simulink model "PASTd"  (R2024b)
settings: Solver=VariableStepAuto  StartTime=0.0  StopTime=10.0  RelTol=1e-3
model workspace (MAT data in the model file):
  w0 = 1
undefined symbols (not defined in the file or in its folder): magnitude
libraries: matrix_library x2
settings Model: ParameterArgumentNames=w0  Creator=yingwan  LastModifiedBy=yingwan
settings ConfigComp: CovBoundaryAbsTol=1.0e-5

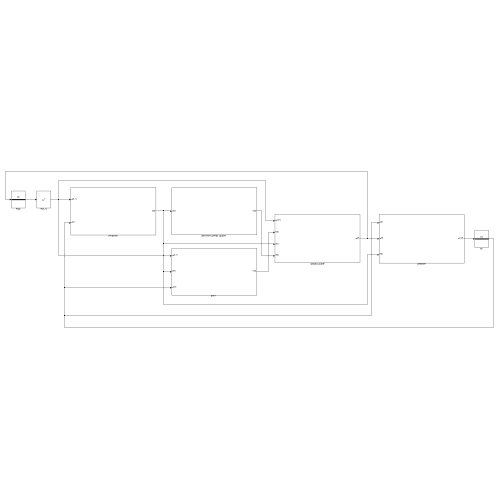
[thumbnail: Simulink's stored preview of the top-level diagram]
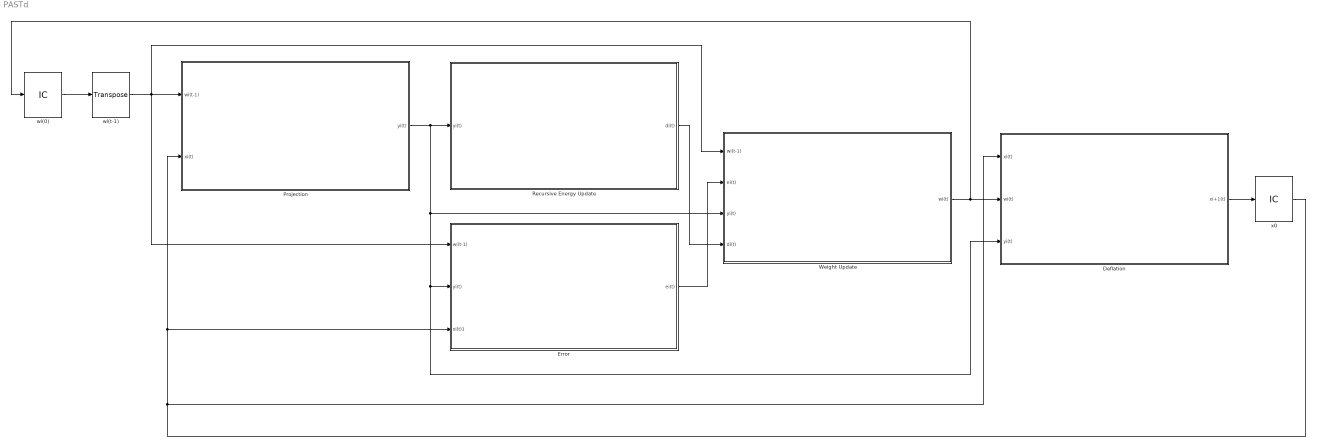
== system PASTd ==
  " Deflation" : Subsystem
  " Weight Update" : Subsystem
  "Error   " : Subsystem
  Projection : Subsystem
  "Recursive Energy Update  " : Subsystem
  wi(0) : InitialCondition
  wi(t-1) : matrix_library/Transpose
  x0 : InitialCondition
  wires:
  Projection/1(yi(t)) -> " Weight Update"/3(yi(t)), " Deflation"/3(yi(t)), "Error   "/2(yi(t)), "Recursive Energy Update  "/1(yi(t))
  wi(t-1)/1 -> "Error   "/1(wi(t-1)), Projection/1(wi(t-1)), " Weight Update"/1(wi(t-1))
  x0/1 -> Projection/2(xi(t)), "Error   "/3(xi(t)1), " Deflation"/1(xi(t))
  " Weight Update"/1(wi(t)) -> wi(0)/1, " Deflation"/2(wi(t))
  "Error   "/1(ei(t)) -> " Weight Update"/2(ei(t))
  "Recursive Energy Update  "/1(di(t)) -> " Weight Update"/4(di(t))
  wi(0)/1 -> wi(t-1)/1
  " Deflation"/1(xi+1(t)) -> x0/1

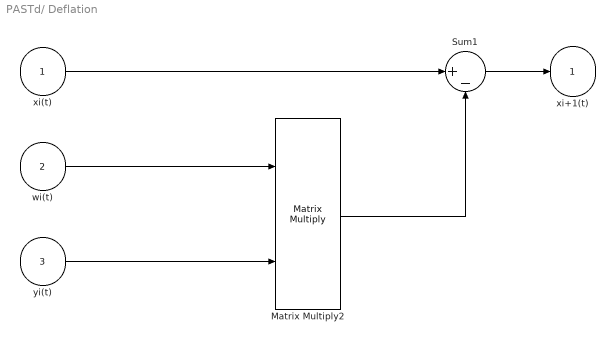
== system PASTd/ Deflation ==
  xi(t) : Inport
  wi(t) : Inport  Port=2
  yi(t) : Inport  Port=3
  Matrix Multiply2 : Product  Multiplication=Matrix(*)
  Sum1 : Sum  Inputs=|+-
  xi+1(t) : Outport
  wires:
  wi(t)/1 -> Matrix Multiply2/1
  yi(t)/1 -> Matrix Multiply2/2
  xi(t)/1 -> Sum1/1
  Matrix Multiply2/1 -> Sum1/2
  Sum1/1 -> xi+1(t)/1

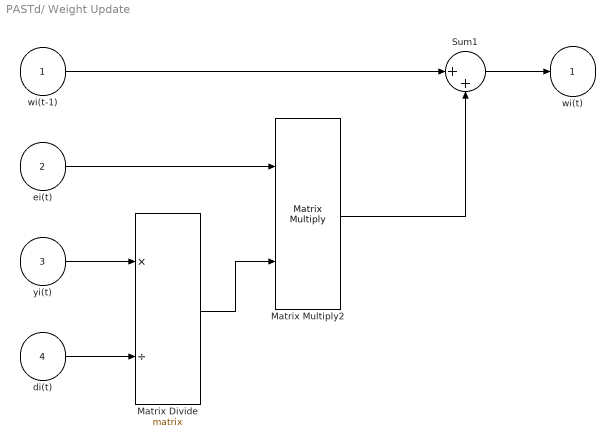
== system PASTd/ Weight Update ==
  wi(t-1) : Inport
  ei(t) : Inport  Port=2
  yi(t) : Inport  Port=3
  di(t) : Inport  Port=4
  Matrix Divide : Product  Inputs=*/  Multiplication=Matrix(*)
  Matrix Multiply2 : Product  Multiplication=Matrix(*)
  Sum1 : Sum  Inputs=|++
  wi(t) : Outport
  wires:
  ei(t)/1 -> Matrix Multiply2/1
  yi(t)/1 -> Matrix Divide/1
  di(t)/1 -> Matrix Divide/2
  Matrix Divide/1 -> Matrix Multiply2/2
  wi(t-1)/1 -> Sum1/1
  Matrix Multiply2/1 -> Sum1/2
  Sum1/1 -> wi(t)/1

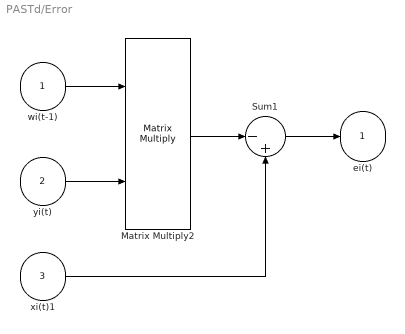
== system PASTd/Error    ==
  wi(t-1) : Inport
  yi(t) : Inport  Port=2
  xi(t)1 : Inport  Port=3
  Matrix Multiply2 : Product  Multiplication=Matrix(*)
  Sum1 : Sum  Inputs=|-+
  ei(t) : Outport
  wires:
  yi(t)/1 -> Matrix Multiply2/2
  wi(t-1)/1 -> Matrix Multiply2/1
  Matrix Multiply2/1 -> Sum1/1
  xi(t)1/1 -> Sum1/2
  Sum1/1 -> ei(t)/1

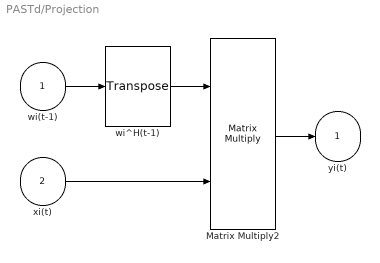
== system PASTd/Projection ==
  wi(t-1) : Inport
  xi(t) : Inport  Port=2
  Matrix Multiply2 : Product  Multiplication=Matrix(*)
  wi^H(t-1) : matrix_library/Transpose
  yi(t) : Outport
  wires:
  xi(t)/1 -> Matrix Multiply2/2
  wi(t-1)/1 -> wi^H(t-1)/1
  wi^H(t-1)/1 -> Matrix Multiply2/1
  Matrix Multiply2/1 -> yi(t)/1

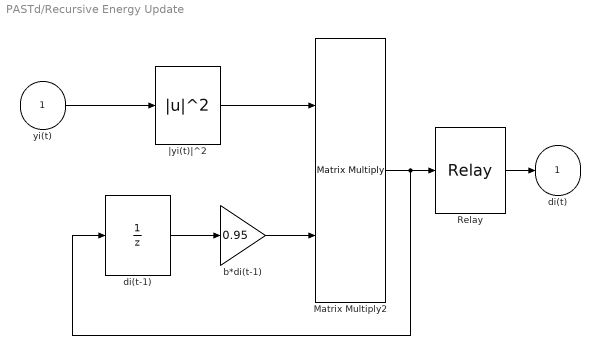
== system PASTd/Recursive Energy Update   ==
  yi(t) : Inport
  Matrix Multiply2 : Product  Multiplication=Matrix(*)
  Relay : Relay
  b*di(t-1) : Gain  Gain=0.95
  di(t-1) : UnitDelay  SampleTime=-1  HasFrameUpgradeWarning=on
  |yi(t)|^2 : Math  Operator=magnitude^2
  di(t) : Outport
  wires:
  Matrix Multiply2/1 -> di(t-1)/1, Relay/1
  |yi(t)|^2/1 -> Matrix Multiply2/1
  yi(t)/1 -> |yi(t)|^2/1
  di(t-1)/1 -> b*di(t-1)/1
  b*di(t-1)/1 -> Matrix Multiply2/2
  Relay/1 -> di(t)/1
